simulink model "nid_motion"  (Simulink 7.6)
settings: Solver=FixedStepDiscrete  StartTime=0.0  StopTime=inf  RelTol=1e-3
libraries: nid_lib x2
settings Model: Creator=tchikama  LastModifiedBy=tchikama
settings DataIOCC: SaveOutput=off
settings OptimizationCC: SimCompilerOptimization=On
settings HardwareCC: ProdIntDivRoundTo=Zero  ProdEndianess=LittleEndian  ProdHWDeviceType=Generic->32-bit x86 compatible
settings RTWCC: ProcessScript=grt_make_rtw_hook  RTWCompilerOptimization=On
settings CodeAppCC: MaxIdLength=95

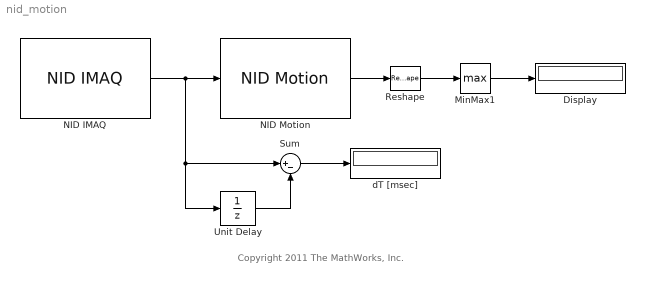
== system nid_motion ==
  note: Copyright 2011 The MathWorks, Inc.
  Display : Display
  MinMax1 : MinMax  Function=max
  NID IMAQ : nid_lib/NID IMAQ  imaq_depth=off  imaq_motion=on  imaq_image=off  view_point=off  imaq_skeleton=off  imaq_ir=off  mirror_image=off  imaq_sample_time=1/30
  NID Motion : nid_lib/NID Motion  viewer=off
  Reshape : Reshape
  Sum : Sum  Inputs=|+-
  Unit Delay : UnitDelay  SampleTime=-1
  dT [msec] : Display
  wires:
  Reshape/1 -> MinMax1/1
  NID IMAQ/1 -> Unit Delay/1, Sum/1, NID Motion/1
  Unit Delay/1 -> Sum/2
  Sum/1 -> dT [msec]/1
  NID Motion/1 -> Reshape/1
  MinMax1/1 -> Display/1
